simulink model "PTSTemperatureDerate"  (R2024b)
settings: Solver=FixedStepAuto  StartTime=0.0  StopTime=10.0  RelTol=1e-3  EnableMultiTasking=on
settings Model: DataDictionary=Master_Dictionary.sldd  EnableAccessToBaseWorkspace=off  Creator=torni  LastModifiedBy=Will
settings OptimizationCC: DefaultParameterBehavior=Inlined  EnhancedBackFolding=on  PassReuseOutputArgsAs=Individual arguments  ZeroExternalMemoryAtStartup=off  ZeroInternalMemoryAtStartup=off  MaxStackSize=8192  OptimizeBlockOrder=speed  DifferentSizesBufferReuse=on  OptimizationCustomize=off  EfficientTunableParamExpr=on
settings DebuggingCC: ParameterTunabilityLossMsg=error
settings HardwareCC: ProdBitPerPointer=32  ProdBitPerSizeT=32  ProdBitPerPtrDiffT=32  ProdLargestAtomicInteger=Long  ProdLargestAtomicFloat=Double  ProdWordSize=32  ProdLongLongMode=on  ProdHWDeviceType=ARM Compatible->ARM Cortex-M
settings SFSimCC: MATLABDynamicMemAlloc=off
settings RTWCC: Description=Embedded Coder  SystemTargetFile=ert.tlc  HardwareBoard=STM32H7xx Based (Single-core)  TemplateMakefile=ert_default_tmf  Toolchain=GNU Tools for ARM Embedded Processors
settings CodeAppCC: ForceParamTrailComments=on  IgnoreCustomStorageClasses=off  OperatorAnnotations=on  SimulinkDataObjDesc=on  SFDataObjDesc=on  InsertBlockDesc=on
settings ERTTargetCC: TargetLangStandard=C99 (ISO)  CodeReplacementLibrary=ARM Cortex-M  ExtModeTransport=3  ExtModeStaticAlloc=on  ExtModeStaticAllocSize=2048  ExtModeMexFile=ext_xcp  ExtModeIntrfLevel=Level2 - Open

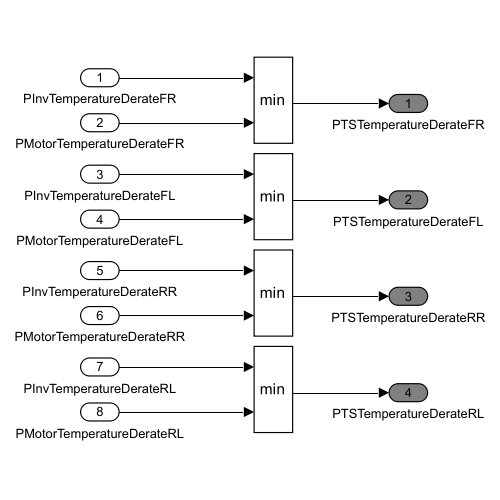
[thumbnail: Simulink's stored preview of the top-level diagram]
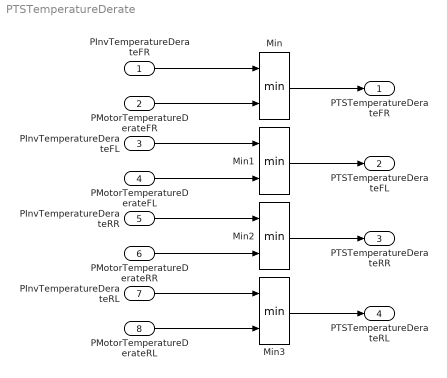
== system PTSTemperatureDerate ==
  PInvTemperatureDerateFR : Inport  OutDataTypeStr=double
  PMotorTemperatureDerateFR : Inport  Port=2  OutDataTypeStr=double
  PInvTemperatureDerateFL : Inport  Port=3  OutDataTypeStr=double
  PMotorTemperatureDerateFL : Inport  Port=4  OutDataTypeStr=double
  PInvTemperatureDerateRR : Inport  Port=5  OutDataTypeStr=double
  PMotorTemperatureDerateRR : Inport  Port=6  OutDataTypeStr=double
  PInvTemperatureDerateRL : Inport  Port=7  OutDataTypeStr=double
  PMotorTemperatureDerateRL : Inport  Port=8  OutDataTypeStr=double
  Min{,1..3} (4 alike) : MinMax  Inputs=2
  PTSTemperatureDerateFR : Outport  OutDataTypeStr=double  VectorParamsAs1DForOutWhenUnconnected=off
  PTSTemperatureDerateFL : Outport  Port=2  OutDataTypeStr=double  VectorParamsAs1DForOutWhenUnconnected=off
  PTSTemperatureDerateRR : Outport  Port=3  OutDataTypeStr=double  VectorParamsAs1DForOutWhenUnconnected=off
  PTSTemperatureDerateRL : Outport  Port=4  OutDataTypeStr=double  VectorParamsAs1DForOutWhenUnconnected=off
  wires:
  Min/1 -> PTSTemperatureDerateFR/1
  PInvTemperatureDerateFR/1 -> Min/1
  PMotorTemperatureDerateFR/1 -> Min/2
  PMotorTemperatureDerateFL/1 -> Min1/2
  PInvTemperatureDerateFL/1 -> Min1/1
  Min1/1 -> PTSTemperatureDerateFL/1
  Min2/1 -> PTSTemperatureDerateRR/1
  PInvTemperatureDerateRR/1 -> Min2/1
  PMotorTemperatureDerateRR/1 -> Min2/2
  PMotorTemperatureDerateRL/1 -> Min3/2
  PInvTemperatureDerateRL/1 -> Min3/1
  Min3/1 -> PTSTemperatureDerateRL/1
